simulink model "NEW_CONTROLLER"  (Simulink 5.0)
settings: Solver=ode45  StartTime=0.0  StopTime=10.0  RelTol=1e-3
settings Model: LastModifiedBy=dev

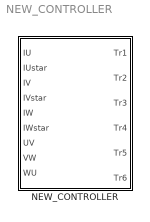
== system NEW_CONTROLLER ==
  NEW_CONTROLLER : Subsystem

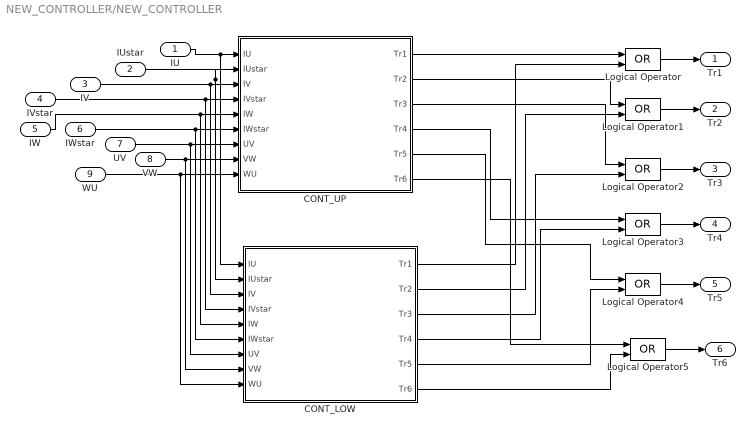
== system NEW_CONTROLLER/NEW_CONTROLLER ==
  IU : Inport
  IUstar : Inport  Port=2
  IV : Inport  Port=3
  IVstar : Inport  Port=4
  IW : Inport  Port=5
  IWstar : Inport  Port=6
  UV : Inport  Port=7
  VW : Inport  Port=8
  WU : Inport  Port=9
  CONT_LOW : Stateflow chart  TreatAsAtomicUnit=on
  CONT_UP : Stateflow chart  TreatAsAtomicUnit=on
  Logical Operator{,1..5} (6 alike) : Logic  Operator=OR  AllPortsSameDT=off
  Tr1 : Outport
  Tr2 : Outport  Port=2
  Tr3 : Outport  Port=3
  Tr4 : Outport  Port=4
  Tr5 : Outport  Port=5
  Tr6 : Outport  Port=6
  wires:
  IU/1 -> CONT_LOW/1(IU), CONT_UP/1(IU)
  IUstar/1 -> CONT_LOW/2(IUstar), CONT_UP/2(IUstar)
  IV/1 -> CONT_LOW/3(IV), CONT_UP/3(IV)
  IVstar/1 -> CONT_LOW/4(IVstar), CONT_UP/4(IVstar)
  IW/1 -> CONT_LOW/5(IW), CONT_UP/5(IW)
  IWstar/1 -> CONT_LOW/6(IWstar), CONT_UP/6(IWstar)
  UV/1 -> CONT_LOW/7(UV), CONT_UP/7(UV)
  VW/1 -> CONT_LOW/8(VW), CONT_UP/8(VW)
  WU/1 -> CONT_UP/9(WU), CONT_LOW/9(WU)
  CONT_UP/1(Tr1) -> Logical Operator/1
  CONT_LOW/1(Tr1) -> Logical Operator/2
  Logical Operator/1 -> Tr1/1
  Logical Operator1/1 -> Tr2/1
  CONT_UP/2(Tr2) -> Logical Operator1/1
  CONT_LOW/2(Tr2) -> Logical Operator1/2
  Logical Operator2/1 -> Tr3/1
  CONT_UP/3(Tr3) -> Logical Operator2/1
  CONT_LOW/3(Tr3) -> Logical Operator2/2
  Logical Operator3/1 -> Tr4/1
  CONT_UP/4(Tr4) -> Logical Operator3/1
  CONT_LOW/4(Tr4) -> Logical Operator3/2
  Logical Operator4/1 -> Tr5/1
  CONT_UP/5(Tr5) -> Logical Operator4/1
  CONT_LOW/5(Tr5) -> Logical Operator4/2
  Logical Operator5/1 -> Tr6/1
  CONT_UP/6(Tr6) -> Logical Operator5/1
  CONT_LOW/6(Tr6) -> Logical Operator5/2

== stateflow chart NEW_CONTROLLER/CONT_LOW ==
  settings: updateMethod=CONTINUOUS  sampleTime=0.0001
  state A/
    state A1/
      during: Tr1=0;Tr3=0;Tr4=0;
      Tr2=0;Tr5=0;Tr6=0;
    state A2/
      during: Tr1=0; Tr3=0; Tr4=0; Tr2=0; Tr5=0;
      Tr6=1;
    (default) -> A1
  state B/
    state B1/
      during: Tr3=0;Tr5=0;Tr4=0;Tr2=0;
      Tr1=0; Tr6=0;
    state B2/
      during:Tr3=0;Tr5=0;Tr4=0;Tr2=0;
      Tr1=0; Tr6=1;
    (default) -> B1
  state C/
    state C1/
      during: Tr3=0;Tr5=0;Tr4=0;Tr2=0;
      Tr1=0; Tr6=0;
    state C2/
      during: Tr3=0;Tr5=0; Tr4=0; Tr6=0;
      Tr1=0; Tr2=1;
    (default) -> C1
  state D/
    state D1/
      during: Tr3=0;Tr5=0;Tr4=0;Tr2=0;
      Tr1=0; Tr6=0;
    state D2/
      during: Tr1=0; Tr5=0;Tr4=0; Tr6=0;
      Tr3=0; Tr2=1;
    (default) -> D1
  state E/
    state E1/
      during: Tr3=0;Tr5=0;Tr4=0;Tr2=0;
      Tr1=0; Tr6=0;
    state E2/
      during: Tr1=0; Tr5=0; Tr6=0; Tr2=0;
      Tr3=0; Tr4=1;
    (default) -> E1
  state F/
    state F1/
      during: Tr3=0;Tr5=0;Tr4=0;Tr2=0;
      Tr1=0; Tr6=0;
    state F2/
      during: Tr1=0; Tr3=0; Tr6=0; Tr2=0;
      Tr5=0; Tr4=1;
    (default) -> F1
  (default) -> A : [1]
  A1 -> A2 : [IV>IVstar]
  A2 -> A1 : [IV<IVstar]
  B1 -> B2 : [IVstar <IV]
  B2 -> B1 : [IVstar>IV]
  A -> B : [WU==1]
  C1 -> C2 : [IWstar<IW]
  C2 -> C1 : [IWstar>IW]
  B -> C : [VW==1]
  D1 -> D2 : [IWstar<IW]
  D2 -> D1 : [IWstar>IW]
  C -> D : [UV==1]
  E1 -> E2 : [IUstar<IU]
  E2 -> E1 : [IUstar>IU]
  D -> E : [WU==1]
  F1 -> F2 : [IUstar<IU]
  F2 -> F1 : [IUstar>IU]
  E -> F : [VW==1]
  F -> A : [UV==1]
  data: IU input double; IUstar input double; IV input double; IVstar input double; IW input double; IWstar input double; Tr1 output double; Tr2 output double; Tr3 output double; Tr4 output double; Tr5 output double; Tr6 output double; UV input double; VW input double; WU input double

== stateflow chart NEW_CONTROLLER/CONT_UP ==
  settings: updateMethod=CONTINUOUS  sampleTime=0.0001
  state A/
    state A11/
      during:Tr1=0;Tr1=0;Tr2=0;Tr3=0;Tr4=0;Tr5=0;
      Tr6=0;
    state A2/
      during: Tr1=0; Tr3=0; Tr4=0; Tr2=0; Tr5=1;
      Tr6=0;
    (default) -> A11
  state B/
    state B1/
      during: Tr3=0;Tr5=0;Tr4=0;Tr2=0;
      Tr1=0; Tr6=0;
    state B2/
      during:Tr3=0;Tr5=0;Tr4=0;Tr2=0;
      Tr1=1; Tr6=0;
    (default) -> B1
  state C/
    state C1/
      during: Tr3=0;Tr5=0;Tr4=0;Tr2=0;
      Tr1=0; Tr6=0;
    state C2/
      during: Tr3=0;Tr5=0; Tr4=0; Tr6=0;
      Tr1=1; Tr2=0;
    (default) -> C1
  state D/
    state D1/
      during: Tr3=0;Tr5=0;Tr4=0;Tr2=0;
      Tr1=0; Tr6=0;
    state D2/
      during: Tr1=0; Tr5=0;Tr4=0; Tr6=0;
      Tr3=1; Tr2=0;
    (default) -> D1
  state E/
    state E1/
      during: Tr3=0;Tr5=0;Tr4=0;Tr2=0;
      Tr1=0; Tr6=0;
    state E2/
      during: Tr1=0; Tr5=0; Tr6=0; Tr2=0;
      Tr3=1; Tr4=0;
    (default) -> E1
  state F/
    state F1/
      during: Tr3=0;Tr5=0;Tr4=0;Tr2=0;
      Tr1=0; Tr6=0;
    state F2/
      during: Tr1=0; Tr3=0; Tr6=0; Tr2=0;
      Tr5=1; Tr4=0;
    (default) -> F1
  A11 -> A2 : [IWstar>IW]
  A2 -> A11 : [IWstar<IW]
  B1 -> B2 : [IU <IUstar]
  B2 -> B1 : [IU>IUstar]
  A -> B : [WU==1]
  C1 -> C2 : [IUstar>IU]
  C2 -> C1 : [IUstar<IU]
  B -> C : [VW==1]
  D1 -> D2 : [IV<IVstar]
  D2 -> D1 : [IV>IVstar]
  C -> D : [UV==1]
  E1 -> E2 : [IVstar>IV]
  E2 -> E1 : [IVstar<IV]
  D -> E : [WU==1]
  F -> A : [UV==1]
  F1 -> F2 : [IW<IWstar]
  F2 -> F1 : [IW>IWstar]
  E -> F : [VW==1]
  (default) -> A : [1]
  data: IU input double; IUstar input double; IV input double; IVstar input double; IW input double; IWstar input double; Tr1 output double; Tr2 output double; Tr3 output double; Tr4 output double; Tr5 output double; Tr6 output double; UV input double; VW input double; WU input double
